simulink model "CL_Simulator"  (R2019b)
settings: Solver=VariableStepAuto  StartTime=0.0  StopTime=10.0  RelTol=1e-3
undefined symbols (not defined in the file or in its folder): ctrller, scenario
settings Model: Creator=akshita_jain  LastModifiedBy=akshita_jain

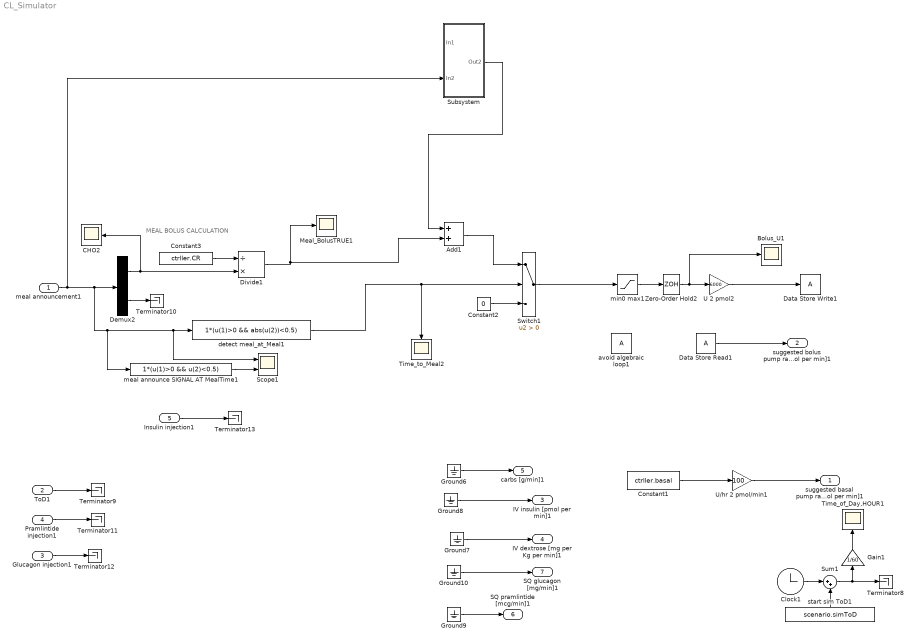
== system CL_Simulator ==
  note: MEAL BOLUS CALCULATION
  meal announcement1 : Inport
  ToD1 : Inport  Port=2
  Glucagon injection1 : Inport  Port=3
  Pramlintide injection1 : Inport  Port=4
  Insulin injection1 : Inport  Port=5
  Add1 : Sum
  Bolus_U1 : Scope
  CHO2 : Scope
  Clock1 : Clock
  Constant1 : Constant  Value=ctrller.basal
  Constant2 : Constant  Value=0
  Constant3 : Constant  Value=ctrller.CR
  Data Store Read1 : DataStoreRead  SampleTime=0
  Data Store Write1 : DataStoreWrite
  Demux2 : Demux  Outputs=2
  Divide1 : Product  Inputs=/*
  Gain1 : Gain  Gain=1/60
  Ground{6..10} (5 alike) : Ground
  Meal_BolusTRUE1 : Scope
  Scope1 : Scope  NumInputPorts=2
  Subsystem : Subsystem
  Sum1 : Sum  Inputs=|++
  Switch1 : Switch  Criteria=u2 > Threshold
  Terminator{8..13} (6 alike) : Terminator
  Time_of_Day,HOUR1 : Scope
  Time_to_Meal2 : Scope
  U 2 pmol2 : Gain  Gain=6000
  U/hr 2 pmol/min1 : Gain  Gain=100
  Zero-Order Hold2 : ZeroOrderHold
  avoid algebraic loop1 : DataStoreMemory  ReadBeforeWriteMsg=warning  WriteAfterWriteMsg=warning  WriteAfterReadMsg=warning  ShowAdditionalParam=off
  detect meal_at_Meal1 : Fcn  Expr=1*(u(1)>0 && abs(u(2))<0.5)
  meal announce SIGNAL AT MealTime1 : Fcn  Expr=1*(u(1)>0 && u(2)<0.5)  SampleTime=1
  min0 max1 : Saturate  UpperLimit=100  LowerLimit=0
  start sim ToD1 : Constant  Value=scenario.simToD
  suggested basal pump rate [pmol per min]1 : Outport
  suggested bolus pump rate [pmol per min]1 : Outport  Port=2
  IV insulin [pmol per min]1 : Outport  Port=3
  IV dextrose [mg per Kg per min]1 : Outport  Port=4
  carbs [g/min]1 : Outport  Port=5
  SQ pramlintide [mcg/min]1 : Outport  Port=6
  SQ glucagon [mg/min]1 : Outport  Port=7
  wires:
  meal announce SIGNAL AT MealTime1/1 -> Scope1/2
  Demux2/2 -> Terminator10/1
  Ground10/1 -> SQ glucagon [mg/min]1/1
  Ground9/1 -> SQ pramlintide [mcg/min]1/1
  Data Store Read1/1 -> suggested bolus pump rate [pmol per min]1/1
  start sim ToD1/1 -> Sum1/2
  Clock1/1 -> Sum1/1
  Sum1/1 -> Terminator8/1, Gain1/1
  Divide1/1 -> Add1/2, Meal_BolusTRUE1/1
  Insulin injection1/1 -> Terminator13/1
  Ground7/1 -> IV dextrose [mg per Kg per min]1/1
  detect meal_at_Meal1/1 -> Switch1/2, Time_to_Meal2/1
  Gain1/1 -> Time_of_Day,HOUR1/1
  Constant3/1 -> Divide1/1
  U/hr 2 pmol/min1/1 -> suggested basal pump rate [pmol per min]1/1
  Constant2/1 -> Switch1/3
  Constant1/1 -> U/hr 2 pmol/min1/1
  Switch1/1 -> min0 max1/1
  Glucagon injection1/1 -> Terminator12/1
  Add1/1 -> Switch1/1
  meal announcement1/1 -> Subsystem/2(In2), Demux2/1, meal announce SIGNAL AT MealTime1/1, detect meal_at_Meal1/1, Scope1/1
  min0 max1/1 -> Zero-Order Hold2/1
  U 2 pmol2/1 -> Data Store Write1/1
  Pramlintide injection1/1 -> Terminator11/1
  ToD1/1 -> Terminator9/1
  Demux2/1 -> Divide1/2, CHO2/1
  Zero-Order Hold2/1 -> U 2 pmol2/1, Bolus_U1/1
  Ground6/1 -> carbs [g/min]1/1
  Ground8/1 -> IV insulin [pmol per min]1/1
  Subsystem/1(Out2) -> Add1/1

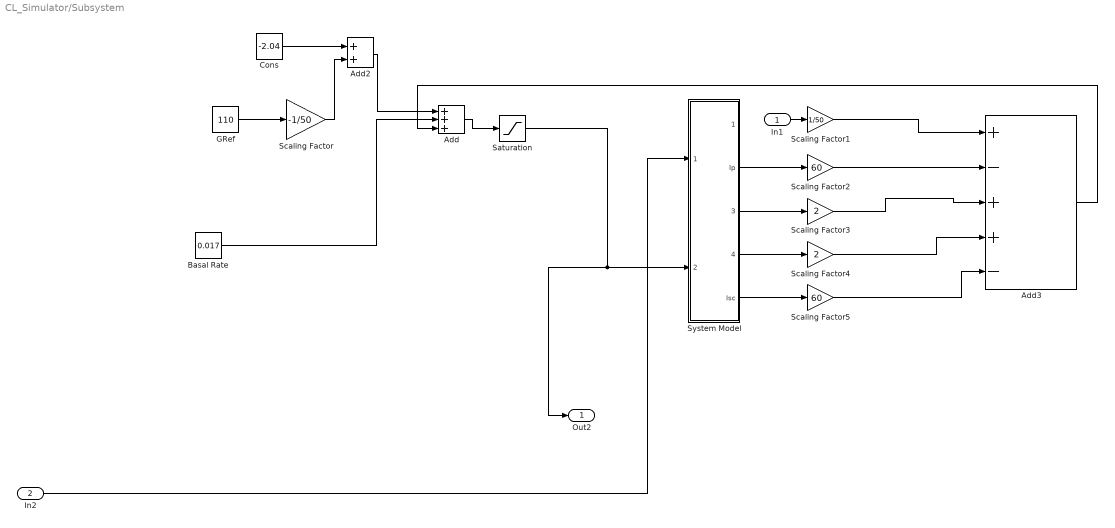
== system CL_Simulator/Subsystem ==
  In1 : Inport
  In2 : Inport  Port=2
  Add : Sum  Inputs=+++
  Add2 : Sum
  Add3 : Sum  Inputs=+-++-
  Basal Rate : Constant  Value=0.017  VectorParams1D=off
  Cons : Constant  Value=-2.04  VectorParams1D=off
  GRef : Constant  Value=110
  Saturation : Saturate  UpperLimit=2  LowerLimit=0
  Scaling Factor : Gain  Gain=-1/50
  Scaling Factor1 : Gain  Gain=1/50
  Scaling Factor2 : Gain  Gain=60
  Scaling Factor3 : Gain  Gain=2
  Scaling Factor4 : Gain  Gain=2
  Scaling Factor5 : Gain  Gain=60
  System Model : Subsystem
  Out2 : Outport
  wires:
  System Model/2(Ip) -> Scaling Factor2/1
  Scaling Factor5/1 -> Add3/5
  System Model/4(CHOs) -> Scaling Factor4/1
  Scaling Factor/1 -> Add2/2
  GRef/1 -> Scaling Factor/1
  System Model/3(CHOd) -> Scaling Factor3/1
  Scaling Factor2/1 -> Add3/2
  Basal Rate/1 -> Add/2
  Scaling Factor1/1 -> Add3/1
  Saturation/1 -> System Model/2(Insulin), Out2/1
  System Model/5(Isc) -> Scaling Factor5/1
  Scaling Factor3/1 -> Add3/3
  Add/1 -> Saturation/1
  Add3/1 -> Add/3
  Add2/1 -> Add/1
  In1/1 -> Scaling Factor1/1
  In2/1 -> System Model/1(CHO Intake)
  Cons/1 -> Add2/1
  Scaling Factor4/1 -> Add3/4

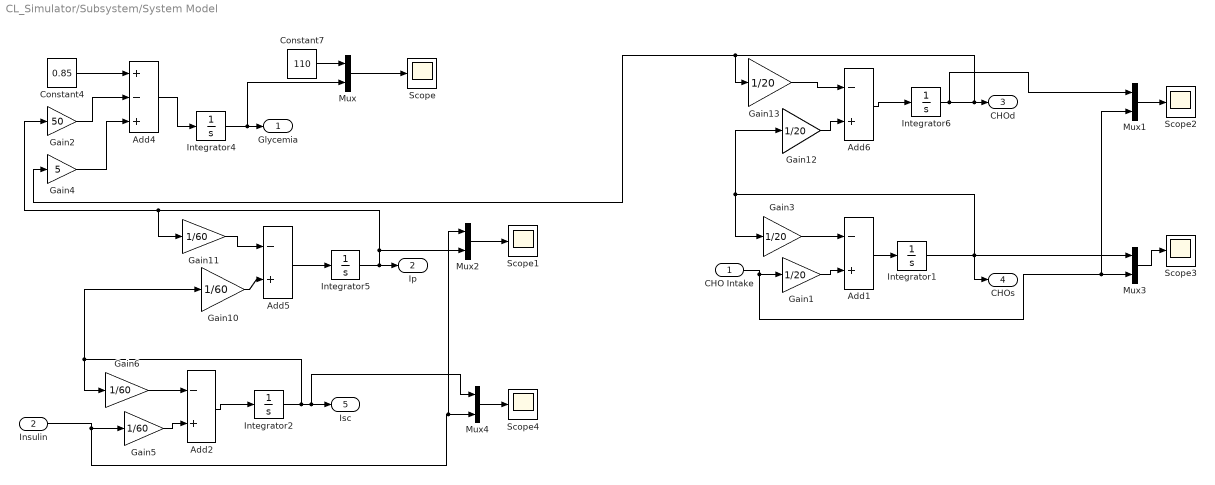
== system CL_Simulator/Subsystem/System Model ==
  CHO Intake : Inport
  Insulin : Inport  Port=2
  Add{1..2,5..6} (4 alike) : Sum  Inputs=-+
  Add4 : Sum  Inputs=+-+
  Constant4 : Constant  Value=0.85  VectorParams1D=off
  Constant7 : Constant  Value=110  VectorParams1D=off
  Gain{1,3,12..13} (4 alike) : Gain  Gain=1/20
  Gain{5..6,10..11} (4 alike) : Gain  Gain=1/60
  Gain2 : Gain  Gain=50
  Gain4 : Gain  Gain=5
  Integrator1 : Integrator  ZeroCross=off
  Integrator2 : Integrator  InitialCondition=0.017  ZeroCross=off
  Integrator4 : Integrator  InitialCondition=110  ZeroCross=off
  Integrator5 : Integrator  InitialCondition=0.017  ZeroCross=off
  Integrator6 : Integrator  ZeroCross=off
  Mux{,1..4} (5 alike) : Mux  Inputs=2
  Scope{,1..4} (5 alike) : Scope
  Glycemia : Outport
  Ip : Outport  Port=2
  CHOd : Outport  Port=3
  CHOs : Outport  Port=4
  Isc : Outport  Port=5
  wires:
  Gain4/1 -> Add4/3
  Constant4/1 -> Add4/1
  Integrator4/1 -> Mux/2, Glycemia/1
  Gain2/1 -> Add4/2
  Add4/1 -> Integrator4/1
  Mux/1 -> Scope/1
  Add5/1 -> Integrator5/1
  Constant7/1 -> Mux/1
  Gain11/1 -> Add5/1
  Mux2/1 -> Scope1/1
  Gain10/1 -> Add5/2
  Integrator2/1 -> Mux4/1, Isc/1, Gain10/1, Gain6/1
  Integrator5/1 -> Gain2/1, Gain11/1, Mux2/2, Ip/1
  Integrator6/1 -> Mux1/1, Gain13/1, Gain4/1, CHOd/1
  Integrator1/1 -> CHOs/1, Mux3/1, Gain12/1, Gain3/1
  Add6/1 -> Integrator6/1
  Gain13/1 -> Add6/1
  Gain12/1 -> Add6/2
  Mux1/1 -> Scope2/1
  CHO Intake/1 -> Gain1/1, Mux1/2, Mux3/2
  Add1/1 -> Integrator1/1
  Gain3/1 -> Add1/1
  Gain1/1 -> Add1/2
  Mux3/1 -> Scope3/1
  Add2/1 -> Integrator2/1
  Gain6/1 -> Add2/1
  Gain5/1 -> Add2/2
  Mux4/1 -> Scope4/1
  Insulin/1 -> Mux2/1, Mux4/2, Gain5/1
